simulink model "ButtonLogic"  (R2023b)
(part 3 of 3)

      (junction 1523) -> exitLow
      (junction 1530) -> (junction 1523) : {send(EXIT,Flow);}
      (junction 1517) -> (junction 1530) [order 1] : [exitDur*1000>=BLU_ExitDtctMin_Tms && ...
          | exitDur*1000 <=BLU_ExitDtctMax_Tms ]
      exitHigh -> (junction 1517) : [hasChangedTo(exitButton,false)]
      (junction 1534) -> (junction 1523)
      (junction 1517) -> (junction 1521) [order 2]
      (junction 1520) -> (junction 1534) : {send(longEXIT,Flow);}
      (junction 1521) -> (junction 1520) [order 1] : [exitDur*1000>=BLU_LngExitDtctMin_Tms && ...
          | exitDur*1000 <=BLU_LngExitDtctMax_Tms ]
      (junction 1533) -> (junction 1534)
      (junction 1521) -> (junction 1524) [order 2]
      (junction 1524) -> (junction 1533)
    state CheckCC [parallel]
      settings: executionOrder=5
      state setHigh
        en:
        DASH_CC_Master_Switch = eButton.pressed;
        en,du:
        ccDur = elapsed(sec);
      state setLow
        en:
        DASH_CC_Master_Switch = eButton.released;
      (default) -> ButtonChecker.CheckCC.setLow
      (junction 1018) -> ButtonChecker.CheckCC.setHigh : [ECU_CC_Feature==1]
      ButtonChecker.CheckCC.setLow -> (junction 1018) : [hasChangedTo(cc,true)]
      (junction 1001) -> ButtonChecker.CheckCC.setLow : {send(CC,Flow);}
      (junction 1589) -> (junction 1001) : [ccDur >=BLU_CCDtctMin_Tms && ...
          | ccDur <=BLU_CCDtctMax_Tms ]
      ButtonChecker.CheckCC.setHigh -> (junction 1589) : [hasChangedTo(cc,false)]
    state CheckResume [parallel]
      settings: executionOrder=6
      state setHigh
        en:
        DASH_Cc_Resume_Switch = eButton.pressed;
        en,du:
        resumeDur = elapsed(sec)
      state setLow
        en:
        DASH_Cc_Resume_Switch = eButton.released;
      (default) -> ButtonChecker.CheckResume.setLow
      ButtonChecker.CheckResume.setLow -> (junction 1021) : [hasChangedTo(resume,true)]
      (junction 1021) -> ButtonChecker.CheckResume.setHigh : [ECU_CC_Feature==1]
      (junction 1582) -> ButtonChecker.CheckResume.setLow : {send(RESUME,Flow);}
      (junction 1580) -> (junction 1582) : [resumeDur >=BLU_ResDtctMin_Tms && ...
          | resumeDur <=BLU_ResDtctMax_Tms ]
      ButtonChecker.CheckResume.setHigh -> (junction 1580) : [hasChangedTo(resume,false)]
    state CheckCCSet [parallel]
      settings: executionOrder=7
      state setHigh
        en:
        DASH_Cc_Set_Switch = eButton.pressed;
      state setLow
        en:
        DASH_Cc_Set_Switch = eButton.released;
      (default) -> ButtonChecker.CheckCCSet.setLow
      ButtonChecker.CheckCCSet.setLow -> (junction 1038) : [hasChangedTo(ccSet,true)]
      (junction 1038) -> ButtonChecker.CheckCCSet.setHigh : [ECU_CC_Feature==1]
      (junction 1039) -> ButtonChecker.CheckCCSet.setLow [commented out] : {send(longCC,Flow);}
      ButtonChecker.CheckCCSet.setHigh -> (junction 1039) [commented out] : [duration(set==true,msec) >=BLU_LngCCDtctMin_Tms && ...
          | duration(set==true,msec) <=BLU_LngCCDtctMax_Tms ]
      (junction 1040) -> ButtonChecker.CheckCCSet.setLow : [hasChangedTo(cc,false)]
          | {send(CCSet,Flow);}
      ButtonChecker.CheckCCSet.setHigh -> (junction 1040) : [duration(set==true,msec) >=BLU_CCSetDtctMin_Tms && ...
          | duration(set==true,msec) <=BLU_CCSetDtctMax_Tms ]
  state startLapOrLapTimer [function]
    (default) -> (junction 97)
  state copyRoundTimeData [function]
    (default) -> (junction 271) : {index  = 0;}
    (junction 271) -> (junction 274) [order 1] : [index<BLU_MaxRndTimeLoopLim]
    (junction 296) -> (junction 271) : {loc_roundTimerData_arr[index] = roundTimerData_arr[index];}
    (junction 271) -> (junction 278) [order 2]
    (junction 274) -> (junction 296) : {index++;}
  state updateRoundTimeData [function]
    (default) -> (junction 285) : {index  = 0;}
    (junction 285) -> (junction 287) [order 1] : [index<BLU_MaxRndTimeLoopLim]
    (junction 298) -> (junction 285) : { rndTimerData_arr[index]= loc_roundTimerData_arr[index];}
    (junction 285) -> (junction 289) [order 2]
    (junction 287) -> (junction 298) : {index++;}
  data: index local double; index local double; set input boolean; up input boolean; down input boolean; DASH_RCM_Set_Switch output Enum: eButton =eButton.released; DASH_RCM_Down_Switch output Enum: eButton =eButton.released; DASH_RCM_Up_Switch output Enum: eButton =eButton.released; DASH_RCM_Exit_Switch output Enum: eButton =eButton.released; exitButton input boolean; ECU_SL_Status parameter; ECU_CC_Feature parameter; DASH_Cc_Resume_Switch output Enum: eButton =eButton.released; DASH_Cc_Set_Switch output Enum: eButton =eButton.released; CCU_RCM_Feature parameter; CCU_RCM_Ready_Status parameter; currentState output Enum: eStateName =eStateName.MAIN_SCREEN; ECU_SL_LED parameter; ECU_SL_Feature parameter; CCU_Status parameter; CCU_TbT_Navigation_Feature parameter; CCU_Music_Feature parameter; Heated_Grips parameter; rideMode output Enum: eRideMode =eRideMode.street; BLU_MaxRndTimeLoopLim parameter; roundTimerData_arr input single size=99; roundTimeCounter output double =0; loc_roundTimerData_arr local single size=99; rndTimerData_arr output single size=99; BLU_UpDtctMax_Tms parameter; BLU_UpDtctMin_Tms parameter; BLU_LngDwnDtctMax_Tms parameter; BLU_LngDwnDtctMin_Tms parameter; BLU_LngExitDtctMax_Tms parameter; BLU_LngExitDtctMin_Tms parameter; BLU_LngSetDtctMax_Tms parameter; BLU_LngSetDtctMin_Tms parameter; ECU_Quickshifter_Feature parameter; BLU_SetDtctMin_Tms parameter; BLU_SetDtctMax_Tms parameter; BLU_LngUpDtctMin_Tms parameter; BLU_LngUpDtctMax_Tms parameter; BLU_ExitDtctMin_Tms parameter; BLU_ExitDtctMax_Tms parameter; BLU_DwnDtctMin_Tms parameter; BLU_DwnDtctMax_Tms parameter; cc input; DASH_CC_Master_Switch output Enum: eButton =eButton.released; BLU_CCDtctMax_Tms parameter; BLU_CCDtctMin_Tms parameter; BLU_ResDtctMax_Tms parameter; BLU_ResDtctMin_Tms parameter; resume input; ccSet input; BLU_CCSetDtctMax_Tms parameter; BLU_CCSetDtctMin_Tms parameter; vehSpeed input; CCU_BT_Status parameter; odoUnits input; exitDur local double; setDur local double; downDur local double; ccDur local double; upDur local double; resumeDur local double; ABS_Launch_Control_Feature parameter; ABS_Mode_Feature parameter; ABS_TC_Mode_Response parameter; ECU_Drive_Mode_Response parameter; DASH_Drive_Mode_Request output uint16 =0; DASH_TC_Mode_Request output uint16 =0; killSwitch input; DASH_ABS_Mode_Request output uint8 =0; ABS_TC_MTC_Mode_Feature parameter; ABS_ABS_Mode_Response parameter; DASH_MTC_Off_Switch output uint16 =0; odoValue input; ShiftLightStatus output uint16 =0; rpm1 output uint16 [5000..11000] =5000; rpm2 output uint16 [5000..11000] =5000; heatedGrips output uint16 =0; quickSelectorDown output uint16 =0; quickSelectorUp output uint16 =0; DASH_RCM_Ready_Switch output uint16; navigationStatus output uint16; QuickSelectorDbg output uint8; HeatedGripsMode local Enum: eHeatedGripsMode =eHeatedGripsMode.OFF; popUpState output uint16; INwarning input; INcall input; INcallEnded input; BLU_BTSearchDur_Tms parameter; btPhoneFound input; jumpDigits local uint8; btPhonePairingError input; btHeadsetPairingError input; btHeadsetFound input; btPhonePassKeyRcvd input; btPhonePrngScs input; phonePaired local boolean =false; headsetPaired local boolean =false; btHdstPrngScs input; DASH_Grip_Installation output uint8 [0..1] =0; HCU_Grip_Heat_Level_Res input; cnfrmAppReg local uint16; rgstrAppReply input; BLU_RND_TMR_LOOP parameter uint8; CCU_Corded_Headset parameter uint8; btPhoneDelErr input; btHdstDelErr input; InCallStatus input; DASH_SL_Switch output; favSlot2Sel local double; favSlot3Sel local double; favSlot4Sel local double; favSlot1Sel local double; IgnBattFlg input
  events: longUP local FUNCTION_CALL_EVENT; UP local FUNCTION_CALL_EVENT; longDOWN local FUNCTION_CALL_EVENT; DOWN local FUNCTION_CALL_EVENT; SET local FUNCTION_CALL_EVENT; EXIT local FUNCTION_CALL_EVENT; longSET local FUNCTION_CALL_EVENT; longEXIT local FUNCTION_CALL_EVENT; CC local FUNCTION_CALL_EVENT; RESUME local FUNCTION_CALL_EVENT; CCSet local FUNCTION_CALL_EVENT; warning local RISING_EDGE_EVENT; incomingCall local RISING_EDGE_EVENT; callEnded local FUNCTION_CALL_EVENT
